simulink model "Xe_Model_Redo_June_26"  (R2018a)
settings: Solver=VariableStepAuto  StartTime=0.0  StopTime=5E5+96*60*60  RelTol=1e-3
values from neighbouring files (symbols this model uses):
  A_pipe = pi*r_pipe^2    (= 0.0126676869774)    [Startup_Script.m]
  alpha_FS = 0.517E-16    (= 5.17e-17)    [Startup_Script.m]
  alpha_G_R1 = 0.334E-17    (= 3.34e-18)    [Startup_Script.m]
  alpha_G_R2 = 0.699E-17    (= 6.99e-18)    [Startup_Script.m]
  alpha_G_R3 = 0.669E-17    (= 6.69e-18)    [Startup_Script.m]
  alpha_G_R4 = 0.791E-18    (= 7.91e-19)    [Startup_Script.m]
  D_g = 2.37E-9    (= 2.37e-09)    [Startup_Script.m]
  epsilon = 0.1    [Startup_Script.m]
  eta_b = 1E-4    (= 0.0001)    [Startup_Script.m]
  eta_fs = 1.2E-4    (= 0.00012)    [Startup_Script.m]
  f_cv = 0.004    [Startup_Script.m]
  FS_Mu_A = 4340    [Startup_Script.m]
  FS_Mu_K = 0.084    [Startup_Script.m]
  FS_Mu_MSRE = 0.007027    [Startup_Script.m]
  FS_rho_A = 3.628    [Startup_Script.m]
  FS_rho_B = 0.00066    [Startup_Script.m]
  FS_rho_MSRE = 2082    [Startup_Script.m]
  gamma_i = 0.0293524    [Startup_Script.m]
  gamma_te = 0.0322482    [Startup_Script.m]
  gamma_xe = 0.00257324    [Startup_Script.m]
  h_fc = 1.6    [Startup_Script.m]
  H_Xe_a = 5.713e-13    [Startup_Script.m]
  H_Xe_b = -7.937e-10    [Startup_Script.m]
  H_Xe_c = 2.809e-07    [Startup_Script.m]
  HX_r_Tube = ((0.5-0.042)/2)*2.54E-2    (= 0.0058166)    [Startup_Script.m]
  HX_XS = HX_N_Tubes*(pi*HX_r_Tube^2)    (= 0.0168999490356)    [Startup_Script.m]
  k_b = 1.3806E-23    (= 1.3806e-23)    [Startup_Script.m]
  lambda_i = 2.9306070546251702E-5    (= 2.93060705463e-05)    [Startup_Script.m]
  lambda_te = 0.036481430555786593    (= 0.0364814305558)    [Startup_Script.m]
  lambda_xe = 2.0924e-05    [Startup_Script.m]
  N_FC_R1 = 12    [Startup_Script.m]
  N_FC_R2 = 940    [Startup_Script.m]
  N_FC_R3 = 108    [Startup_Script.m]
  N_FC_R4 = 78    [Startup_Script.m]
  P_pump = 35420    [Startup_Script.m]
  phi0 = 3.98E+17    (= 3.98e+17)    [Startup_Script.m]
  phi_G_R_1 = mean(interp1(phi_G_R,phi_G_phi, linspace(0,r_g_r1)))    [Startup_Script.m]
  phi_G_R_2 = mean(interp1(phi_G_R,phi_G_phi, linspace(r_g_r1,r_g_r2)))    [Startup_Script.m]
  phi_G_R_3 = mean(interp1(phi_G_R,phi_G_phi, linspace(r_g_r2,r_g_r3)))    [Startup_Script.m]
  phi_G_R_4 = mean(interp1(phi_G_R,phi_G_phi, linspace(r_g_r3,r_g_r4)))    [Startup_Script.m]
  Q_strpr = 0.003155    [Startup_Script.m]
  Q_tot = 0.07571    [Startup_Script.m]
  r_b = 0.000254    [Startup_Script.m]
  r_fc = 0.79e-2    (= 0.0079)    [Startup_Script.m]
  r_pipe = (5E-2*2.54)/2    (= 0.0635)    [Startup_Script.m]
  r_xe = 2.16E-10    (= 2.16e-10)    [Startup_Script.m]
  Re_CA = 25800    [Startup_Script.m]
  Re_LH = 1E4    (= 10000)    [Startup_Script.m]
  Re_UH = 1E4    (= 10000)    [Startup_Script.m]
  sig_a_xe = 1.18E-22    (= 1.18e-22)    [Startup_Script.m]
  Sig_f = 0.15    [Startup_Script.m]
  T_CA_0 = T_INLET    (= 907.594444444)    [Startup_Script.m]
  T_FP_0 = T_OUTLET    (= 935.372222222)    [Startup_Script.m]
  T_FS_R_1_0 = mean(interp1(R_fs_m,T_fs_K, linspace(0,r_g_r1)))    [Startup_Script.m]
  T_FS_R_2_0 = mean(interp1(R_fs_m,T_fs_K, linspace(r_g_r1,r_g_r2)))    [Startup_Script.m]
  T_FS_R_3_0 = mean(interp1(R_fs_m,T_fs_K, linspace(r_g_r2,r_g_r3)))    [Startup_Script.m]
  T_FS_R_4_0 = mean(interp1(R_fs_m,T_fs_K, linspace(r_g_r3,r_g_r4)))    [Startup_Script.m]
  T_G_R_1_0 = mean(interp1(R_gr_m,T_gr_K, linspace(0,r_g_r1)))    [Startup_Script.m]
  T_HX_0 = 0.5*(T_OUTLET + T_INLET)    (= 921.483333333)    [Startup_Script.m]
  T_LH_0 = T_INLET    (= 907.594444444)    [Startup_Script.m]
  T_Mes = 928.15    [Startup_Script.m]
  T_P100_0 = T_OUTLET    (= 935.372222222)    [Startup_Script.m]
  T_P101_0 = T_OUTLET    (= 935.372222222)    [Startup_Script.m]
  T_P102_0 = T_INLET    (= 907.594444444)    [Startup_Script.m]
  T_Salt_0 = 900    [Startup_Script.m]
  T_UH_0 = T_OUTLET    (= 935.372222222)    [Startup_Script.m]
  U_FC_R1 = 0.607    [Startup_Script.m]
  U_FC_R2 = 0.183    [Startup_Script.m]
  U_FC_R3 = 0.454    [Startup_Script.m]
  U_FC_R4 = 0.250    (= 0.25)    [Startup_Script.m]
  V_CA_0 = 9.7*cubed_foot_to_cubed_meter    (= 0.274673445)    [Startup_Script.m]
  V_FP_0 = (0.9+3.2)*cubed_foot_to_cubed_meter    (= 0.116099085)    [Startup_Script.m]
  V_HX_0 = 6.1*cubed_foot_to_cubed_meter    (= 0.172732785)    [Startup_Script.m]
  V_LH_0 = 10.0*cubed_foot_to_cubed_meter    (= 0.2831685)    [Startup_Script.m]
  V_P100_0 = 2.1*cubed_foot_to_cubed_meter    (= 0.059465385)    [Startup_Script.m]
  V_P101_0 = 0.8*cubed_foot_to_cubed_meter    (= 0.02265348)    [Startup_Script.m]
  V_P102_0 = 2.2*cubed_foot_to_cubed_meter    (= 0.06229707)    [Startup_Script.m]
  V_R1_0 = V_Core_FS_0 *N_FC_R1/N_FC_tot    (= 0.00753107712766)    [Startup_Script.m]
  V_R2_0 = V_Core_FS_0 *N_FC_R2/N_FC_tot    (= 0.589934375)    [Startup_Script.m]
  V_R3_0 = V_Core_FS_0 *N_FC_R3/N_FC_tot    (= 0.0677796941489)    [Startup_Script.m]
  V_R4_0 = V_Core_FS_0 *N_FC_R4/N_FC_tot    (= 0.0489520013298)    [Startup_Script.m]
  V_UH_0 = 10.5*cubed_foot_to_cubed_meter    (= 0.297326925)    [Startup_Script.m]
undefined symbols (not defined in the file or in its folder): magnitude, V_CA, V_HX, V_P2, V_P3, V_R1, V_R2, V_R3, V_R4, V_UH
libraries: simulink x4, dspindex x4, dspstat3 x4, SignalEditorBlockLib x2
(part 6 of 11)

== system Xe_Model_Redo_June_26/Bubbles/Bubble Mass Transfer/P100/KMA_P100/Pipe Bubble  MTC ==
  note: ORNL-TM-2245 p. 23 - eqn 36
  note: Thermophysical Properties
  U : Inport
  T : Inport  Port=2
  r : Inport  Port=3
  Constant : Constant  Value=0.0096
  Constant1 : Constant  Value=0.913
  Constant2 : Constant  Value=0.346
  Constant4 : Constant
  Density W Scaling1 : Subsystem
  Divide1 : Product  Inputs=*/
  Gain : Gain  Gain=2
  Mass Diffusion Coeffecient [m^2 /s] : Subsystem
  Math Function : Math  Operator=pow  SaturateOnIntegerOverflow=on
  Math Function1 : Math  Operator=pow  SaturateOnIntegerOverflow=on
  Product : Product
  Reynolds Number : Subsystem
  Schmidt Number : Subsystem
  Sherwood Number : Product  Inputs=4
  Viscosity W Scaling1 : Subsystem
  k_m_b : Outport
  wires:
  Constant1/1 -> Math Function/2
  Gain/1 -> Divide1/2, Reynolds Number/4(L)
  Constant2/1 -> Math Function1/2
  [D_FS_Local] -> Divide1/1
  Constant4/1 -> Sherwood Number/3
  Constant/1 -> Sherwood Number/1
  Divide1/1 -> Product/2
  Math Function1/1 -> Sherwood Number/4
  Schmidt Number/1(Sc) -> Math Function1/1
  Math Function/1 -> Sherwood Number/2
  Sherwood Number/1 -> Product/1
  Product/1 -> k_m_b/1
  Reynolds Number/1(Re) -> Math Function/1
  U/1 -> Reynolds Number/1(Flow_Velocity)
  [Mu_FS_Local] -> Schmidt Number/1(mu)
  [Rho_FS_Local] -> Schmidt Number/2(rho)
  [D_FS_Local] -> Schmidt Number/3(D)
  [Mu_FS_Local] -> Reynolds Number/2(mu)
  [Rho_FS_Local] -> Reynolds Number/3(rho)
  r/1 -> Gain/1
  T/1 -> Mass Diffusion Coeffecient [m^2 /s]/2(T_Salt [k]), Viscosity W Scaling1/1(T_Salt [k]), Density W Scaling1/1(T_Salt [k])
  Density W Scaling1/1(rho_FS [kg/m^3]) -> [Rho_FS_Local]
  Viscosity W Scaling1/1(mu [Pa-s]) -> Mass Diffusion Coeffecient [m^2 /s]/1(Mu), [Mu_FS_Local]
  Mass Diffusion Coeffecient [m^2 /s]/1(D [m^2/s]) -> [D_FS_Local]

== system Xe_Model_Redo_June_26/Bubbles/Bubble Mass Transfer/P101/HRT*C_B /Calc H_Xe ==
  T_Salt [K] : Inport
  Constant : Constant  Value=H_Xe_c
  Math Function : Math  Operator=magnitude^2  SaturateOnIntegerOverflow=on
  Sum1 : Sum  Inputs=+++
  a const : Gain  Gain=H_Xe_a
  b const : Gain  Gain=H_Xe_b
  H_Xe [m^-3 Pa^-1] : Outport
  wires:
  Sum1/1 -> H_Xe [m^-3 Pa^-1]/1
  a const/1 -> Sum1/1
  Constant/1 -> Sum1/3
  b const/1 -> Sum1/2
  Math Function/1 -> a const/1
  T_Salt [K]/1 -> b const/1, Math Function/1

== system Xe_Model_Redo_June_26/Bubbles/Bubble Mass Transfer/P101/KMA_P101/CA  CV Area ==
  Node Vol. : Inport
  CV Vol to Mass Transfer Area1 : Subsystem
  A : Outport
  wires:
  CV Vol to Mass Transfer Area1/1(A) -> A/1
  Node Vol./1 -> CV Vol to Mass Transfer Area1/1(V)

== system Xe_Model_Redo_June_26/Bubbles/Bubble Mass Transfer/P101/KMA_P101/Pipe Bubble  MTC ==
  note: ORNL-TM-2245 p. 23 - eqn 36
  note: Thermophysical Properties
  U : Inport
  T : Inport  Port=2
  r : Inport  Port=3
  Constant : Constant  Value=0.0096
  Constant1 : Constant  Value=0.913
  Constant2 : Constant  Value=0.346
  Constant4 : Constant
  Density W Scaling1 : Subsystem
  Divide1 : Product  Inputs=*/
  Gain : Gain  Gain=2
  Mass Diffusion Coeffecient [m^2 /s] : Subsystem
  Math Function : Math  Operator=pow  SaturateOnIntegerOverflow=on
  Math Function1 : Math  Operator=pow  SaturateOnIntegerOverflow=on
  Product : Product
  Reynolds Number : Subsystem
  Schmidt Number : Subsystem
  Sherwood Number : Product  Inputs=4
  Viscosity W Scaling1 : Subsystem
  k_m_b : Outport
  wires:
  Constant1/1 -> Math Function/2
  r/1 -> Gain/1
  Constant2/1 -> Math Function1/2
  [D_FS_Local] -> Divide1/1
  Constant4/1 -> Sherwood Number/3
  Constant/1 -> Sherwood Number/1
  Divide1/1 -> Product/2
  Math Function1/1 -> Sherwood Number/4
  Schmidt Number/1(Sc) -> Math Function1/1
  Math Function/1 -> Sherwood Number/2
  Sherwood Number/1 -> Product/1
  Product/1 -> k_m_b/1
  Reynolds Number/1(Re) -> Math Function/1
  U/1 -> Reynolds Number/1(Flow_Velocity)
  [Mu_FS_Local] -> Schmidt Number/1(mu)
  [Rho_FS_Local] -> Schmidt Number/2(rho)
  [D_FS_Local] -> Schmidt Number/3(D)
  [Mu_FS_Local] -> Reynolds Number/2(mu)
  [Rho_FS_Local] -> Reynolds Number/3(rho)
  T/1 -> Mass Diffusion Coeffecient [m^2 /s]/2(T_Salt [k]), Viscosity W Scaling1/1(T_Salt [k]), Density W Scaling1/1(T_Salt [k])
  Density W Scaling1/1(rho_FS [kg/m^3]) -> [Rho_FS_Local]
  Viscosity W Scaling1/1(mu [Pa-s]) -> Mass Diffusion Coeffecient [m^2 /s]/1(Mu), [Mu_FS_Local]
  Mass Diffusion Coeffecient [m^2 /s]/1(D [m^2/s]) -> [D_FS_Local]
  Gain/1 -> Divide1/2, Reynolds Number/4(L)

== system Xe_Model_Redo_June_26/Bubbles/Bubble Mass Transfer/P102/HRT*C_B /Calc H_Xe ==
  T_Salt [K] : Inport
  Constant : Constant  Value=H_Xe_c
  Math Function : Math  Operator=magnitude^2  SaturateOnIntegerOverflow=on
  Sum1 : Sum  Inputs=+++
  a const : Gain  Gain=H_Xe_a
  b const : Gain  Gain=H_Xe_b
  H_Xe [m^-3 Pa^-1] : Outport
  wires:
  Sum1/1 -> H_Xe [m^-3 Pa^-1]/1
  a const/1 -> Sum1/1
  Constant/1 -> Sum1/3
  b const/1 -> Sum1/2
  Math Function/1 -> a const/1
  T_Salt [K]/1 -> b const/1, Math Function/1

== system Xe_Model_Redo_June_26/Bubbles/Bubble Mass Transfer/P102/KMA_P102/CA  CV Area ==
  Node Vol. : Inport
  CV Vol to Mass Transfer Area1 : Subsystem
  A : Outport
  wires:
  CV Vol to Mass Transfer Area1/1(A) -> A/1
  Node Vol./1 -> CV Vol to Mass Transfer Area1/1(V)

== system Xe_Model_Redo_June_26/Bubbles/Bubble Mass Transfer/P102/KMA_P102/Pipe Bubble  MTC ==
  note: NB: this is supposed to be for the pipe
  note: ORNL-TM-2245 p. 23 - eqn 36
  note: Thermophysical Properties
  U : Inport
  T : Inport  Port=2
  r : Inport  Port=3
  Constant : Constant  Value=0.0096
  Constant1 : Constant  Value=0.913
  Constant2 : Constant  Value=0.346
  Constant4 : Constant
  Density W Scaling1 : Subsystem
  Divide1 : Product  Inputs=*/
  Gain : Gain  Gain=2
  Mass Diffusion Coeffecient [m^2 /s] : Subsystem
  Math Function : Math  Operator=pow  SaturateOnIntegerOverflow=on
  Math Function1 : Math  Operator=pow  SaturateOnIntegerOverflow=on
  Product : Product
  Reynolds Number : Subsystem
  Schmidt Number : Subsystem
  Sherwood Number : Product  Inputs=4
  Viscosity W Scaling1 : Subsystem
  k_m_b : Outport
  wires:
  Constant1/1 -> Math Function/2
  r/1 -> Gain/1
  Constant2/1 -> Math Function1/2
  [D_FS_Local] -> Divide1/1
  Constant4/1 -> Sherwood Number/3
  Constant/1 -> Sherwood Number/1
  Divide1/1 -> Product/2
  Math Function1/1 -> Sherwood Number/4
  Schmidt Number/1(Sc) -> Math Function1/1
  Math Function/1 -> Sherwood Number/2
  Sherwood Number/1 -> Product/1
  Product/1 -> k_m_b/1
  Reynolds Number/1(Re) -> Math Function/1
  U/1 -> Reynolds Number/1(Flow_Velocity)
  [Mu_FS_Local] -> Schmidt Number/1(mu)
  [Rho_FS_Local] -> Schmidt Number/2(rho)
  [D_FS_Local] -> Schmidt Number/3(D)
  [Mu_FS_Local] -> Reynolds Number/2(mu)
  [Rho_FS_Local] -> Reynolds Number/3(rho)
  T/1 -> Mass Diffusion Coeffecient [m^2 /s]/2(T_Salt [k]), Viscosity W Scaling1/1(T_Salt [k]), Density W Scaling1/1(T_Salt [k])
  Density W Scaling1/1(rho_FS [kg/m^3]) -> [Rho_FS_Local]
  Viscosity W Scaling1/1(mu [Pa-s]) -> Mass Diffusion Coeffecient [m^2 /s]/1(Mu), [Mu_FS_Local]
  Mass Diffusion Coeffecient [m^2 /s]/1(D [m^2/s]) -> [D_FS_Local]
  Gain/1 -> Divide1/2, Reynolds Number/4(L)

== system Xe_Model_Redo_June_26/Bubbles/Bubble Mass Transfer/UH/HRT*C_B /Calc H_Xe ==
  T_Salt [K] : Inport
  Constant : Constant  Value=H_Xe_c
  Math Function : Math  Operator=magnitude^2  SaturateOnIntegerOverflow=on
  Sum1 : Sum  Inputs=+++
  a const : Gain  Gain=H_Xe_a
  b const : Gain  Gain=H_Xe_b
  H_Xe [m^-3 Pa^-1] : Outport
  wires:
  Sum1/1 -> H_Xe [m^-3 Pa^-1]/1
  a const/1 -> Sum1/1
  Constant/1 -> Sum1/3
  b const/1 -> Sum1/2
  Math Function/1 -> a const/1
  T_Salt [K]/1 -> b const/1, Math Function/1

== system Xe_Model_Redo_June_26/Bubbles/Bubble Mass Transfer/UH/KMA_UH/CA  CV Area ==
  Node Vol. : Inport
  CV Vol to Mass Transfer Area1 : Subsystem
  A : Outport
  wires:
  CV Vol to Mass Transfer Area1/1(A) -> A/1
  Node Vol./1 -> CV Vol to Mass Transfer Area1/1(V)

== system Xe_Model_Redo_June_26/Bubbles/Bubble Mass Transfer/UH/KMA_UH/MTC UH ==
  note: Perry's P. 5-69
  note: Thermophysical Properties
  T : Inport
  Constant : Constant  Value=1.0
  Constant1 : Constant  Value=1/3
  Constant2 : Constant  Value=1/3
  Constant3 : Constant  Value=Re_UH
  Constant4 : Constant
  Density W Scaling1 : Subsystem
  Divide1 : Product  Inputs=*/
  Gain : Gain  Gain=2
  Mass Diffusion Coeffecient [m^2 /s]1 : Subsystem
  Math Function : Math  Operator=pow  SaturateOnIntegerOverflow=on
  Math Function1 : Math  Operator=pow  SaturateOnIntegerOverflow=on
  Product : Product
  Re_Num  Scaled : Subsystem
  Schmidt Number : Subsystem
  Sherwood Number : Product  Inputs=4
  Viscosity W Scaling1 : Subsystem
  k_m_b : Outport
  wires:
  Constant1/1 -> Math Function/2
  Constant2/1 -> Math Function1/2
  [D_FS_Local] -> Divide1/1
  Constant4/1 -> Sherwood Number/3
  Constant/1 -> Sherwood Number/1
  Divide1/1 -> Product/2
  Math Function1/1 -> Sherwood Number/4
  Schmidt Number/1(Sc) -> Math Function1/1
  Math Function/1 -> Sherwood Number/2
  Sherwood Number/1 -> Product/1
  Product/1 -> k_m_b/1
  Re_Num  Scaled/1(Re) -> Math Function/1
  [Mu_FS_Local] -> Schmidt Number/1(mu)
  [Rho_FS_Local] -> Schmidt Number/2(rho)
  [D_FS_Local] -> Schmidt Number/3(D)
  T/1 -> Mass Diffusion Coeffecient [m^2 /s]1/2(T_Salt [k]), Viscosity W Scaling1/1(T_Salt [k]), Density W Scaling1/1(T_Salt [k]), Re_Num  Scaled/1(T)
  Density W Scaling1/1(rho_FS [kg/m^3]) -> [Rho_FS_Local]
  Viscosity W Scaling1/1(mu [Pa-s]) -> Mass Diffusion Coeffecient [m^2 /s]1/1(Mu), [Mu_FS_Local]
  Mass Diffusion Coeffecient [m^2 /s]1/1(D [m^2/s]) -> [D_FS_Local]
  Constant3/1 -> Re_Num  Scaled/2(Re_0)
  [r_b] -> Gain/1
  Gain/1 -> Divide1/2

== system Xe_Model_Redo_June_26/Graphite /Graphite Region 1/Graphite MTC R1/Density W Scaling/Cantor F1 Density ==
  note: K -> deg. C
  T_Salt [k] : Inport
  Constant : Constant  Value=FS_rho_A
  Constant1 : Constant  Value=FS_rho_B
  Constant2 : Constant  Value=273.15
  Display : Display
      settings: Format=short_e
  Display1 : Display
  Product : Product
  Sum : Sum  Inputs=|+-
  Sum1 : Sum  Inputs=+-
  "g/cm^3 -> kg/m^3" : Gain  Gain=1000
  rho [kg/m^3] : Outport
  wires:
  Sum/1 -> "g/cm^3 -> kg/m^3"/1
  Product/1 -> Sum/2
  Constant1/1 -> Display/1, Product/1
  "g/cm^3 -> kg/m^3"/1 -> rho [kg/m^3]/1
  Constant/1 -> Display1/1, Sum/1
  T_Salt [k]/1 -> Sum1/1
  Constant2/1 -> Sum1/2
  Sum1/1 -> Product/2

== system Xe_Model_Redo_June_26/Graphite /Graphite Region 1/Graphite MTC R1/Density W Scaling/Cantor F1 Density1 ==
  note: K -> deg. C
  T_Salt [k] : Inport
  Constant : Constant  Value=FS_rho_A
  Constant1 : Constant  Value=FS_rho_B
  Constant2 : Constant  Value=273.15
  Display : Display
      settings: Format=short_e
  Display1 : Display
  Product : Product
  Sum : Sum  Inputs=|+-
  Sum1 : Sum  Inputs=+-
  "g/cm^3 -> kg/m^3" : Gain  Gain=1000
  rho [kg/m^3] : Outport
  wires:
  Sum/1 -> "g/cm^3 -> kg/m^3"/1
  Product/1 -> Sum/2
  Constant1/1 -> Display/1, Product/1
  "g/cm^3 -> kg/m^3"/1 -> rho [kg/m^3]/1
  Constant/1 -> Display1/1, Sum/1
  T_Salt [k]/1 -> Sum1/1
  Constant2/1 -> Sum1/2
  Sum1/1 -> Product/2

== system Xe_Model_Redo_June_26/Graphite /Graphite Region 1/Graphite MTC R1/Viscosity W Scaling/Cantor Viscosity F1 ==
  T_Salt [k] : Inport
  Constant : Constant  Value=FS_Mu_A
  Constant1 : Constant  Value=FS_Mu_K
  Display1 : Display
  Divide : Product  Inputs=*/
  Math Function : Math  SaturateOnIntegerOverflow=on
  Product : Product
  "centipoise -> Pa S" : Gain  Gain=0.001
  Mu [Pa S] : Outport
  wires:
  Constant1/1 -> Product/2
  T_Salt [k]/1 -> Divide/2
  "centipoise -> Pa S"/1 -> Display1/1, Mu [Pa S]/1
  Product/1 -> "centipoise -> Pa S"/1
  Constant/1 -> Divide/1
  Math Function/1 -> Product/1
  Divide/1 -> Math Function/1

== system Xe_Model_Redo_June_26/Graphite /Graphite Region 1/Graphite MTC R1/Viscosity W Scaling/Nominal Value for Cantor Viscosity F1 ==
  T_Salt [k] : Inport
  Constant : Constant  Value=FS_Mu_A
  Constant1 : Constant  Value=FS_Mu_K
  Display1 : Display
  Divide : Product  Inputs=*/
  Math Function : Math  SaturateOnIntegerOverflow=on
  Product : Product
  "centipoise -> Pa S" : Gain  Gain=0.001
  Mu [Pa S] : Outport
  wires:
  Constant1/1 -> Product/2
  T_Salt [k]/1 -> Divide/2
  "centipoise -> Pa S"/1 -> Display1/1, Mu [Pa S]/1
  Product/1 -> "centipoise -> Pa S"/1
  Constant/1 -> Divide/1
  Math Function/1 -> Product/1
  Divide/1 -> Math Function/1

== system Xe_Model_Redo_June_26/Graphite /Graphite Region 1/Graphite Stringer/Calc Flux/Calc H_Xe ==
  T_Salt [K] : Inport
  Constant : Constant  Value=H_Xe_c
  Math Function : Math  Operator=magnitude^2  SaturateOnIntegerOverflow=on
  Sum1 : Sum  Inputs=+++
  a const : Gain  Gain=H_Xe_a
  b const : Gain  Gain=H_Xe_b
  H_Xe [m^-3 Pa^-1] : Outport
  wires:
  Sum1/1 -> H_Xe [m^-3 Pa^-1]/1
  a const/1 -> Sum1/1
  Constant/1 -> Sum1/3
  b const/1 -> Sum1/2
  Math Function/1 -> a const/1
  T_Salt [K]/1 -> b const/1, Math Function/1

== system Xe_Model_Redo_June_26/Graphite /Graphite Region 1/Graphite Stringer/HMat/Calc H_Xe ==
  T_Salt [K] : Inport
  Constant : Constant  Value=H_Xe_c
  Math Function : Math  Operator=magnitude^2  SaturateOnIntegerOverflow=on
  Sum1 : Sum  Inputs=+++
  a const : Gain  Gain=H_Xe_a
  b const : Gain  Gain=H_Xe_b
  H_Xe [m^-3 Pa^-1] : Outport
  wires:
  Sum1/1 -> H_Xe [m^-3 Pa^-1]/1
  a const/1 -> Sum1/1
  Constant/1 -> Sum1/3
  b const/1 -> Sum1/2
  Math Function/1 -> a const/1
  T_Salt [K]/1 -> b const/1, Math Function/1

== system Xe_Model_Redo_June_26/Graphite /Graphite Region 1/Lumped Parameter Graphite Model/Subsystem/HRT over epsilon ==
  T : Inport
  Calc H_Xe : Subsystem
  Divide2 : Product  Inputs=***/
  Out1 : Outport
  wires:
  T/1 -> Calc H_Xe/1(T_Salt [K]), Divide2/3
  [epsilon] -> Divide2/4
  Calc H_Xe/1(H_Xe [m^-3 Pa^-1]) -> Divide2/1
  [R_gas] -> Divide2/2
  Divide2/1 -> Out1/1

== system Xe_Model_Redo_June_26/Graphite /Graphite Region 2/Graphite MTC R1/Density W Scaling/Cantor F1 Density ==
  note: K -> deg. C
  T_Salt [k] : Inport
  Constant : Constant  Value=FS_rho_A
  Constant1 : Constant  Value=FS_rho_B
  Constant2 : Constant  Value=273.15
  Display : Display
      settings: Format=short_e
  Display1 : Display
  Product : Product
  Sum : Sum  Inputs=|+-
  Sum1 : Sum  Inputs=+-
  "g/cm^3 -> kg/m^3" : Gain  Gain=1000
  rho [kg/m^3] : Outport
  wires:
  Sum/1 -> "g/cm^3 -> kg/m^3"/1
  Product/1 -> Sum/2
  Constant1/1 -> Display/1, Product/1
  "g/cm^3 -> kg/m^3"/1 -> rho [kg/m^3]/1
  Constant/1 -> Display1/1, Sum/1
  T_Salt [k]/1 -> Sum1/1
  Constant2/1 -> Sum1/2
  Sum1/1 -> Product/2

== system Xe_Model_Redo_June_26/Graphite /Graphite Region 2/Graphite MTC R1/Density W Scaling/Cantor F1 Density1 ==
  note: K -> deg. C
  T_Salt [k] : Inport
  Constant : Constant  Value=FS_rho_A
  Constant1 : Constant  Value=FS_rho_B
  Constant2 : Constant  Value=273.15
  Display : Display
      settings: Format=short_e
  Display1 : Display
  Product : Product
  Sum : Sum  Inputs=|+-
  Sum1 : Sum  Inputs=+-
  "g/cm^3 -> kg/m^3" : Gain  Gain=1000
  rho [kg/m^3] : Outport
  wires:
  Sum/1 -> "g/cm^3 -> kg/m^3"/1
  Product/1 -> Sum/2
  Constant1/1 -> Display/1, Product/1
  "g/cm^3 -> kg/m^3"/1 -> rho [kg/m^3]/1
  Constant/1 -> Display1/1, Sum/1
  T_Salt [k]/1 -> Sum1/1
  Constant2/1 -> Sum1/2
  Sum1/1 -> Product/2

== system Xe_Model_Redo_June_26/Graphite /Graphite Region 2/Graphite MTC R1/Viscosity W Scaling/Cantor Viscosity F1 ==
  T_Salt [k] : Inport
  Constant : Constant  Value=FS_Mu_A
  Constant1 : Constant  Value=FS_Mu_K
  Display1 : Display
  Divide : Product  Inputs=*/
  Math Function : Math  SaturateOnIntegerOverflow=on
  Product : Product
  "centipoise -> Pa S" : Gain  Gain=0.001
  Mu [Pa S] : Outport
  wires:
  Constant1/1 -> Product/2
  T_Salt [k]/1 -> Divide/2
  "centipoise -> Pa S"/1 -> Display1/1, Mu [Pa S]/1
  Product/1 -> "centipoise -> Pa S"/1
  Constant/1 -> Divide/1
  Math Function/1 -> Product/1
  Divide/1 -> Math Function/1

== system Xe_Model_Redo_June_26/Graphite /Graphite Region 2/Graphite MTC R1/Viscosity W Scaling/Nominal Value for Cantor Viscosity F1 ==
  T_Salt [k] : Inport
  Constant : Constant  Value=FS_Mu_A
  Constant1 : Constant  Value=FS_Mu_K
  Display1 : Display
  Divide : Product  Inputs=*/
  Math Function : Math  SaturateOnIntegerOverflow=on
  Product : Product
  "centipoise -> Pa S" : Gain  Gain=0.001
  Mu [Pa S] : Outport
  wires:
  Constant1/1 -> Product/2
  T_Salt [k]/1 -> Divide/2
  "centipoise -> Pa S"/1 -> Display1/1, Mu [Pa S]/1
  Product/1 -> "centipoise -> Pa S"/1
  Constant/1 -> Divide/1
  Math Function/1 -> Product/1
  Divide/1 -> Math Function/1

== system Xe_Model_Redo_June_26/Graphite /Graphite Region 2/Graphite Stringer/Calc Flux/Calc H_Xe ==
  T_Salt [K] : Inport
  Constant : Constant  Value=H_Xe_c
  Math Function : Math  Operator=magnitude^2  SaturateOnIntegerOverflow=on
  Sum1 : Sum  Inputs=+++
  a const : Gain  Gain=H_Xe_a
  b const : Gain  Gain=H_Xe_b
  H_Xe [m^-3 Pa^-1] : Outport
  wires:
  Sum1/1 -> H_Xe [m^-3 Pa^-1]/1
  a const/1 -> Sum1/1
  Constant/1 -> Sum1/3
  b const/1 -> Sum1/2
  Math Function/1 -> a const/1
  T_Salt [K]/1 -> b const/1, Math Function/1

== system Xe_Model_Redo_June_26/Graphite /Graphite Region 2/Graphite Stringer/HMat/Calc H_Xe ==
  T_Salt [K] : Inport
  Constant : Constant  Value=H_Xe_c
  Math Function : Math  Operator=magnitude^2  SaturateOnIntegerOverflow=on
  Sum1 : Sum  Inputs=+++
  a const : Gain  Gain=H_Xe_a
  b const : Gain  Gain=H_Xe_b
  H_Xe [m^-3 Pa^-1] : Outport
  wires:
  Sum1/1 -> H_Xe [m^-3 Pa^-1]/1
  a const/1 -> Sum1/1
  Constant/1 -> Sum1/3
  b const/1 -> Sum1/2
  Math Function/1 -> a const/1
  T_Salt [K]/1 -> b const/1, Math Function/1

== system Xe_Model_Redo_June_26/Graphite /Graphite Region 3/Graphite MTC R1/Density W Scaling/Cantor F1 Density ==
  note: K -> deg. C
  T_Salt [k] : Inport
  Constant : Constant  Value=FS_rho_A
  Constant1 : Constant  Value=FS_rho_B
  Constant2 : Constant  Value=273.15
  Display : Display
      settings: Format=short_e
  Display1 : Display
  Product : Product
  Sum : Sum  Inputs=|+-
  Sum1 : Sum  Inputs=+-
  "g/cm^3 -> kg/m^3" : Gain  Gain=1000
  rho [kg/m^3] : Outport
  wires:
  Sum/1 -> "g/cm^3 -> kg/m^3"/1
  Product/1 -> Sum/2
  Constant1/1 -> Display/1, Product/1
  "g/cm^3 -> kg/m^3"/1 -> rho [kg/m^3]/1
  Constant/1 -> Display1/1, Sum/1
  T_Salt [k]/1 -> Sum1/1
  Constant2/1 -> Sum1/2
  Sum1/1 -> Product/2

== system Xe_Model_Redo_June_26/Graphite /Graphite Region 3/Graphite MTC R1/Density W Scaling/Cantor F1 Density1 ==
  note: K -> deg. C
  T_Salt [k] : Inport
  Constant : Constant  Value=FS_rho_A
  Constant1 : Constant  Value=FS_rho_B
  Constant2 : Constant  Value=273.15
  Display : Display
      settings: Format=short_e
  Display1 : Display
  Product : Product
  Sum : Sum  Inputs=|+-
  Sum1 : Sum  Inputs=+-
  "g/cm^3 -> kg/m^3" : Gain  Gain=1000
  rho [kg/m^3] : Outport
  wires:
  Sum/1 -> "g/cm^3 -> kg/m^3"/1
  Product/1 -> Sum/2
  Constant1/1 -> Display/1, Product/1
  "g/cm^3 -> kg/m^3"/1 -> rho [kg/m^3]/1
  Constant/1 -> Display1/1, Sum/1
  T_Salt [k]/1 -> Sum1/1
  Constant2/1 -> Sum1/2
  Sum1/1 -> Product/2

== system Xe_Model_Redo_June_26/Graphite /Graphite Region 3/Graphite MTC R1/Viscosity W Scaling/Cantor Viscosity F1 ==
  T_Salt [k] : Inport
  Constant : Constant  Value=FS_Mu_A
  Constant1 : Constant  Value=FS_Mu_K
  Display1 : Display
  Divide : Product  Inputs=*/
  Math Function : Math  SaturateOnIntegerOverflow=on
  Product : Product
  "centipoise -> Pa S" : Gain  Gain=0.001
  Mu [Pa S] : Outport
  wires:
  Constant1/1 -> Product/2
  T_Salt [k]/1 -> Divide/2
  "centipoise -> Pa S"/1 -> Display1/1, Mu [Pa S]/1
  Product/1 -> "centipoise -> Pa S"/1
  Constant/1 -> Divide/1
  Math Function/1 -> Product/1
  Divide/1 -> Math Function/1

== system Xe_Model_Redo_June_26/Graphite /Graphite Region 3/Graphite MTC R1/Viscosity W Scaling/Nominal Value for Cantor Viscosity F1 ==
  T_Salt [k] : Inport
  Constant : Constant  Value=FS_Mu_A
  Constant1 : Constant  Value=FS_Mu_K
  Display1 : Display
  Divide : Product  Inputs=*/
  Math Function : Math  SaturateOnIntegerOverflow=on
  Product : Product
  "centipoise -> Pa S" : Gain  Gain=0.001
  Mu [Pa S] : Outport
  wires:
  Constant1/1 -> Product/2
  T_Salt [k]/1 -> Divide/2
  "centipoise -> Pa S"/1 -> Display1/1, Mu [Pa S]/1
  Product/1 -> "centipoise -> Pa S"/1
  Constant/1 -> Divide/1
  Math Function/1 -> Product/1
  Divide/1 -> Math Function/1

== system Xe_Model_Redo_June_26/Graphite /Graphite Region 3/Graphite Stringer/Calc Flux/Calc H_Xe ==
  T_Salt [K] : Inport
  Constant : Constant  Value=H_Xe_c
  Math Function : Math  Operator=magnitude^2  SaturateOnIntegerOverflow=on
  Sum1 : Sum  Inputs=+++
  a const : Gain  Gain=H_Xe_a
  b const : Gain  Gain=H_Xe_b
  H_Xe [m^-3 Pa^-1] : Outport
  wires:
  Sum1/1 -> H_Xe [m^-3 Pa^-1]/1
  a const/1 -> Sum1/1
  Constant/1 -> Sum1/3
  b const/1 -> Sum1/2
  Math Function/1 -> a const/1
  T_Salt [K]/1 -> b const/1, Math Function/1

== system Xe_Model_Redo_June_26/Graphite /Graphite Region 3/Graphite Stringer/HMat/Calc H_Xe ==
  T_Salt [K] : Inport
  Constant : Constant  Value=H_Xe_c
  Math Function : Math  Operator=magnitude^2  SaturateOnIntegerOverflow=on
  Sum1 : Sum  Inputs=+++
  a const : Gain  Gain=H_Xe_a
  b const : Gain  Gain=H_Xe_b
  H_Xe [m^-3 Pa^-1] : Outport
  wires:
  Sum1/1 -> H_Xe [m^-3 Pa^-1]/1
  a const/1 -> Sum1/1
  Constant/1 -> Sum1/3
  b const/1 -> Sum1/2
  Math Function/1 -> a const/1
  T_Salt [K]/1 -> b const/1, Math Function/1

== system Xe_Model_Redo_June_26/Graphite /Graphite Region 4/Graphite MTC R1/Density W Scaling/Cantor F1 Density ==
  note: K -> deg. C
  T_Salt [k] : Inport
  Constant : Constant  Value=FS_rho_A
  Constant1 : Constant  Value=FS_rho_B
  Constant2 : Constant  Value=273.15
  Display : Display
      settings: Format=short_e
  Display1 : Display
  Product : Product
  Sum : Sum  Inputs=|+-
  Sum1 : Sum  Inputs=+-
  "g/cm^3 -> kg/m^3" : Gain  Gain=1000
  rho [kg/m^3] : Outport
  wires:
  Sum/1 -> "g/cm^3 -> kg/m^3"/1
  Product/1 -> Sum/2
  Constant1/1 -> Display/1, Product/1
  "g/cm^3 -> kg/m^3"/1 -> rho [kg/m^3]/1
  Constant/1 -> Display1/1, Sum/1
  T_Salt [k]/1 -> Sum1/1
  Constant2/1 -> Sum1/2
  Sum1/1 -> Product/2

== system Xe_Model_Redo_June_26/Graphite /Graphite Region 4/Graphite MTC R1/Density W Scaling/Cantor F1 Density1 ==
  note: K -> deg. C
  T_Salt [k] : Inport
  Constant : Constant  Value=FS_rho_A
  Constant1 : Constant  Value=FS_rho_B
  Constant2 : Constant  Value=273.15
  Display : Display
      settings: Format=short_e
  Display1 : Display
  Product : Product
  Sum : Sum  Inputs=|+-
  Sum1 : Sum  Inputs=+-
  "g/cm^3 -> kg/m^3" : Gain  Gain=1000
  rho [kg/m^3] : Outport
  wires:
  Sum/1 -> "g/cm^3 -> kg/m^3"/1
  Product/1 -> Sum/2
  Constant1/1 -> Display/1, Product/1
  "g/cm^3 -> kg/m^3"/1 -> rho [kg/m^3]/1
  Constant/1 -> Display1/1, Sum/1
  T_Salt [k]/1 -> Sum1/1
  Constant2/1 -> Sum1/2
  Sum1/1 -> Product/2

== system Xe_Model_Redo_June_26/Graphite /Graphite Region 4/Graphite MTC R1/Viscosity W Scaling/Cantor Viscosity F1 ==
  T_Salt [k] : Inport
  Constant : Constant  Value=FS_Mu_A
  Constant1 : Constant  Value=FS_Mu_K
  Display1 : Display
  Divide : Product  Inputs=*/
  Math Function : Math  SaturateOnIntegerOverflow=on
  Product : Product
  "centipoise -> Pa S" : Gain  Gain=0.001
  Mu [Pa S] : Outport
  wires:
  Constant1/1 -> Product/2
  T_Salt [k]/1 -> Divide/2
  "centipoise -> Pa S"/1 -> Display1/1, Mu [Pa S]/1
  Product/1 -> "centipoise -> Pa S"/1
  Constant/1 -> Divide/1
  Math Function/1 -> Product/1
  Divide/1 -> Math Function/1

== system Xe_Model_Redo_June_26/Graphite /Graphite Region 4/Graphite MTC R1/Viscosity W Scaling/Nominal Value for Cantor Viscosity F1 ==
  T_Salt [k] : Inport
  Constant : Constant  Value=FS_Mu_A
  Constant1 : Constant  Value=FS_Mu_K
  Display1 : Display
  Divide : Product  Inputs=*/
  Math Function : Math  SaturateOnIntegerOverflow=on
  Product : Product
  "centipoise -> Pa S" : Gain  Gain=0.001
  Mu [Pa S] : Outport
  wires:
  Constant1/1 -> Product/2
  T_Salt [k]/1 -> Divide/2
  "centipoise -> Pa S"/1 -> Display1/1, Mu [Pa S]/1
  Product/1 -> "centipoise -> Pa S"/1
  Constant/1 -> Divide/1
  Math Function/1 -> Product/1
  Divide/1 -> Math Function/1

== system Xe_Model_Redo_June_26/Graphite /Graphite Region 4/Graphite Stringer/Calc Flux/Calc H_Xe ==
  T_Salt [K] : Inport
  Constant : Constant  Value=H_Xe_c
  Math Function : Math  Operator=magnitude^2  SaturateOnIntegerOverflow=on
  Sum1 : Sum  Inputs=+++
  a const : Gain  Gain=H_Xe_a
  b const : Gain  Gain=H_Xe_b
  H_Xe [m^-3 Pa^-1] : Outport
  wires:
  Sum1/1 -> H_Xe [m^-3 Pa^-1]/1
  a const/1 -> Sum1/1
  Constant/1 -> Sum1/3
  b const/1 -> Sum1/2
  Math Function/1 -> a const/1
  T_Salt [K]/1 -> b const/1, Math Function/1

== system Xe_Model_Redo_June_26/Graphite /Graphite Region 4/Graphite Stringer/HMat/Calc H_Xe ==
  T_Salt [K] : Inport
  Constant : Constant  Value=H_Xe_c
  Math Function : Math  Operator=magnitude^2  SaturateOnIntegerOverflow=on
  Sum1 : Sum  Inputs=+++
  a const : Gain  Gain=H_Xe_a
  b const : Gain  Gain=H_Xe_b
  H_Xe [m^-3 Pa^-1] : Outport
  wires:
  Sum1/1 -> H_Xe [m^-3 Pa^-1]/1
  a const/1 -> Sum1/1
  Constant/1 -> Sum1/3
  b const/1 -> Sum1/2
  Math Function/1 -> a const/1
  T_Salt [K]/1 -> b const/1, Math Function/1

== system Xe_Model_Redo_June_26/Bubbles/Bubble Mass Transfer/Bubble Total KMA/HX KMA/CA  CV Area/CV Vol to Mass Transfer Area1 ==
  V : Inport
  Divide1 : Product  Inputs=*/
  Product3 : Product
  A : Outport
  wires:
  V/1 -> Divide1/1
  Divide1/1 -> Product3/2
  [V_1_B] -> Divide1/2
  [A_1_B] -> Product3/1
  Product3/1 -> A/1

== system Xe_Model_Redo_June_26/Bubbles/Bubble Mass Transfer/Bubble Total KMA/HX KMA/CA  CV Area/Calc CV Vol W Temp ==
  note: Total CV Vol
  Vol. Gas : Inport
  T : Inport  Port=2
  Constant1 : Constant  Value=T_Salt_0
  Divide : Product  Inputs=**/
  Product : Product
  Product1 : Product
  Subtract1 : Sum  Inputs=+-
  Sum1 : Sum
  vol to num atoms1 : Subsystem
  V Gas : Outport
  wires:
  Product/1 -> Sum1/1, vol to num atoms1/1(vol)
  vol to num atoms1/1(N mols) -> Divide/1
  Product1/1 -> Sum1/2
  T/1 -> Subtract1/1
  Constant1/1 -> Subtract1/2
  Sum1/1 -> V Gas/1
  Vol. Gas/1 -> Product/2
  [R_gas] -> Divide/2
  [P_sys] -> Divide/3
  Divide/1 -> Product1/1
  Subtract1/1 -> Product1/2
  [f_cv_0] -> Product/1

== system Xe_Model_Redo_June_26/Bubbles/Bubble Mass Transfer/Bubble Total KMA/HX KMA/Pipe Buble MTC1/Density W Scaling1 ==
  T_Salt [k] : Inport
  Cantor F1 Density : Subsystem
  Cantor F1 Density1 : Subsystem
  Constant3 : Constant  Value=T_Mes
  Constant4 : Constant  Value=FS_rho_MSRE
  Divide1 : Product  Inputs=*/
  Product1 : Product
  rho_FS [kg/m^3] : Outport
  wires:
  Divide1/1 -> Product1/2
  Cantor F1 Density1/1(rho [kg/m^3]) -> Divide1/2
  Constant4/1 -> Product1/1
  Cantor F1 Density/1(rho [kg/m^3]) -> Divide1/1
  Product1/1 -> rho_FS [kg/m^3]/1
  Constant3/1 -> Cantor F1 Density1/1(T_Salt [k])
  T_Salt [k]/1 -> Cantor F1 Density/1(T_Salt [k])

== system Xe_Model_Redo_June_26/Bubbles/Bubble Mass Transfer/Bubble Total KMA/HX KMA/Pipe Buble MTC1/Mass Diffusion Coeffecient [m^2 //s] ==
  Mu : Inport
  T_Salt [k] : Inport  Port=2
  Constant : Constant  Value=k_b
  Constant1 : Constant  Value=6*pi
  Constant2 : Constant  Value=r_xe
  Divide : Product  Inputs=*/
  Product : Product
  Product1 : Product  Inputs=3
  D [m^2/s] : Outport
  wires:
  Constant1/1 -> Product1/1
  Constant2/1 -> Product1/3
  T_Salt [k]/1 -> Product/1
  Product1/1 -> Divide/2
  Constant/1 -> Product/2
  Product/1 -> Divide/1
  Divide/1 -> D [m^2/s]/1
  Mu/1 -> Product1/2

== system Xe_Model_Redo_June_26/Bubbles/Bubble Mass Transfer/Bubble Total KMA/HX KMA/Pipe Buble MTC1/Reynolds Number ==
  Flow_Velocity : Inport
  mu : Inport  Port=2
  rho : Inport  Port=3
  L : Inport  Port=4
  Divide : Product  Inputs=***/
  Re : Outport
  wires:
  mu/1 -> Divide/4
  rho/1 -> Divide/1
  Divide/1 -> Re/1
  Flow_Velocity/1 -> Divide/2
  L/1 -> Divide/3

== system Xe_Model_Redo_June_26/Bubbles/Bubble Mass Transfer/Bubble Total KMA/HX KMA/Pipe Buble MTC1/Reynolds Number1 ==
  Flow_Velocity [m/s] : Inport
  rho [kg/m^3] : Inport  Port=2
  mu [Pa s] : Inport  Port=3
  Divide : Product  Inputs=***/
  Re : Outport
  wires:
  mu [Pa s]/1 -> Divide/4
  rho [kg/m^3]/1 -> Divide/1
  Divide/1 -> Re/1
  Flow_Velocity [m/s]/1 -> Divide/2
  [r_fc] -> Divide/3

== system Xe_Model_Redo_June_26/Bubbles/Bubble Mass Transfer/Bubble Total KMA/HX KMA/Pipe Buble MTC1/Schmidt Number ==
  mu : Inport
  rho : Inport  Port=2
  D : Inport  Port=3
  Product : Product  Inputs=*//
  Sc : Outport
  wires:
  Product/1 -> Sc/1
  D/1 -> Product/3
  mu/1 -> Product/1
  rho/1 -> Product/2

== system Xe_Model_Redo_June_26/Bubbles/Bubble Mass Transfer/Bubble Total KMA/HX KMA/Pipe Buble MTC1/Schmidt Number1 ==
  mu [Pa s] : Inport
  rho [kg/m^3] : Inport  Port=2
  D [m^2/s] : Inport  Port=3
  Product : Product  Inputs=*//
  Sc : Outport
  wires:
  Product/1 -> Sc/1
  D [m^2/s]/1 -> Product/3
  mu [Pa s]/1 -> Product/1
  rho [kg/m^3]/1 -> Product/2

== system Xe_Model_Redo_June_26/Bubbles/Bubble Mass Transfer/Bubble Total KMA/HX KMA/Pipe Buble MTC1/Viscosity W Scaling1 ==
  T_Salt [k] : Inport
  Cantor Viscosity F1 : Subsystem
  Constant3 : Constant  Value=T_Mes
  Constant4 : Constant  Value=FS_Mu_MSRE
  Divide1 : Product  Inputs=*/
  Nominal Value for Cantor Viscosity F1 : Subsystem
  Product1 : Product
  mu [Pa-s] : Outport
  wires:
  Nominal Value for Cantor Viscosity F1/1(Mu [Pa S]) -> Divide1/2
  Divide1/1 -> Product1/2
  Cantor Viscosity F1/1(Mu [Pa S]) -> Divide1/1
  Product1/1 -> mu [Pa-s]/1
  Constant4/1 -> Product1/1
  Constant3/1 -> Nominal Value for Cantor Viscosity F1/1(T_Salt [k])
  T_Salt [k]/1 -> Cantor Viscosity F1/1(T_Salt [k])

== system Xe_Model_Redo_June_26/Bubbles/Bubble Mass Transfer/Bubble Total KMA/KMA FP/CA  CV Area/CV Vol to Mass Transfer Area1 ==
  V : Inport
  Divide1 : Product  Inputs=*/
  Product3 : Product
  A : Outport
  wires:
  V/1 -> Divide1/1
  Divide1/1 -> Product3/2
  [V_1_B] -> Divide1/2
  [A_1_B] -> Product3/1
  Product3/1 -> A/1

== system Xe_Model_Redo_June_26/Bubbles/Bubble Mass Transfer/Bubble Total KMA/KMA FP/CA  CV Area/Calc CV Vol W Temp ==
  note: Total CV Vol
  Vol. Gas : Inport
  T : Inport  Port=2
  Constant1 : Constant  Value=T_Salt_0
  Divide : Product  Inputs=**/
  Product : Product
  Product1 : Product
  Subtract1 : Sum  Inputs=+-
  Sum1 : Sum
  vol to num atoms1 : Subsystem
  V Gas : Outport
  wires:
  Product/1 -> Sum1/1, vol to num atoms1/1(vol)
  vol to num atoms1/1(N mols) -> Divide/1
  Product1/1 -> Sum1/2
  T/1 -> Subtract1/1
  Constant1/1 -> Subtract1/2
  Sum1/1 -> V Gas/1
  Vol. Gas/1 -> Product/2
  [R_gas] -> Divide/2
  [P_sys] -> Divide/3
  Divide/1 -> Product1/1
  Subtract1/1 -> Product1/2
  [f_cv_0] -> Product/1

== system Xe_Model_Redo_June_26/Bubbles/Bubble Mass Transfer/Bubble Total KMA/KMA FP/Pump Bowl MTC1/Density W Scaling1 ==
  T_Salt [k] : Inport
  Cantor F1 Density : Subsystem
  Cantor F1 Density1 : Subsystem
  Constant3 : Constant  Value=T_Mes
  Constant4 : Constant  Value=FS_rho_MSRE
  Divide1 : Product  Inputs=*/
  Product1 : Product
  rho_FS [kg/m^3] : Outport
  wires:
  Divide1/1 -> Product1/2
  Cantor F1 Density1/1(rho [kg/m^3]) -> Divide1/2
  Constant4/1 -> Product1/1
  Cantor F1 Density/1(rho [kg/m^3]) -> Divide1/1
  Product1/1 -> rho_FS [kg/m^3]/1
  Constant3/1 -> Cantor F1 Density1/1(T_Salt [k])
  T_Salt [k]/1 -> Cantor F1 Density/1(T_Salt [k])

== system Xe_Model_Redo_June_26/Bubbles/Bubble Mass Transfer/Bubble Total KMA/KMA FP/Pump Bowl MTC1/Mass Diffusion Coeffecient [m^2 //s] ==
  Mu : Inport
  T_Salt [k] : Inport  Port=2
  Constant : Constant  Value=k_b
  Constant1 : Constant  Value=6*pi
  Constant2 : Constant  Value=r_xe
  Divide : Product  Inputs=*/
  Product : Product
  Product1 : Product  Inputs=3
  D [m^2/s] : Outport
  wires:
  Constant1/1 -> Product1/1
  Constant2/1 -> Product1/3
  T_Salt [k]/1 -> Product/1
  Product1/1 -> Divide/2
  Constant/1 -> Product/2
  Product/1 -> Divide/1
  Divide/1 -> D [m^2/s]/1
  Mu/1 -> Product1/2

== system Xe_Model_Redo_June_26/Bubbles/Bubble Mass Transfer/Bubble Total KMA/KMA FP/Pump Bowl MTC1/Schmidt Number1 ==
  mu [Pa s] : Inport
  rho [kg/m^3] : Inport  Port=2
  D [m^2/s] : Inport  Port=3
  Product : Product  Inputs=*//
  Sc : Outport
  wires:
  Product/1 -> Sc/1
  D [m^2/s]/1 -> Product/3
  mu [Pa s]/1 -> Product/1
  rho [kg/m^3]/1 -> Product/2

== system Xe_Model_Redo_June_26/Bubbles/Bubble Mass Transfer/Bubble Total KMA/KMA FP/Pump Bowl MTC1/Viscosity W Scaling1 ==
  T_Salt [k] : Inport
  Cantor Viscosity F1 : Subsystem
  Constant3 : Constant  Value=T_Mes
  Constant4 : Constant  Value=FS_Mu_MSRE
  Divide1 : Product  Inputs=*/
  Nominal Value for Cantor Viscosity F1 : Subsystem
  Product1 : Product
  mu [Pa-s] : Outport
  wires:
  Nominal Value for Cantor Viscosity F1/1(Mu [Pa S]) -> Divide1/2
  Divide1/1 -> Product1/2
  Cantor Viscosity F1/1(Mu [Pa S]) -> Divide1/1
  Product1/1 -> mu [Pa-s]/1
  Constant4/1 -> Product1/1
  Constant3/1 -> Nominal Value for Cantor Viscosity F1/1(T_Salt [k])
  T_Salt [k]/1 -> Cantor Viscosity F1/1(T_Salt [k])

== system Xe_Model_Redo_June_26/Bubbles/Bubble Mass Transfer/Bubble Total KMA/KMA_CA/CA  CV Area/CV Vol to Mass Transfer Area1 ==
  V : Inport
  Divide1 : Product  Inputs=*/
  Product3 : Product
  A : Outport
  wires:
  V/1 -> Divide1/1
  Divide1/1 -> Product3/2
  [V_1_B] -> Divide1/2
  [A_1_B] -> Product3/1
  Product3/1 -> A/1

== system Xe_Model_Redo_June_26/Bubbles/Bubble Mass Transfer/Bubble Total KMA/KMA_CA/CA  CV Area/Calc CV Vol W Temp ==
  note: Total CV Vol
  Vol. Gas : Inport
  T : Inport  Port=2
  Constant1 : Constant  Value=T_Salt_0
  Divide : Product  Inputs=**/
  Product : Product
  Product1 : Product
  Subtract1 : Sum  Inputs=+-
  Sum1 : Sum
  vol to num atoms1 : Subsystem
  V Gas : Outport
  wires:
  Product/1 -> Sum1/1, vol to num atoms1/1(vol)
  vol to num atoms1/1(N mols) -> Divide/1
  Product1/1 -> Sum1/2
  T/1 -> Subtract1/1
  Constant1/1 -> Subtract1/2
  Sum1/1 -> V Gas/1
  Vol. Gas/1 -> Product/2
  [R_gas] -> Divide/2
  [P_sys] -> Divide/3
  Divide/1 -> Product1/1
  Subtract1/1 -> Product1/2
  [f_cv_0] -> Product/1

== system Xe_Model_Redo_June_26/Bubbles/Bubble Mass Transfer/Bubble Total KMA/KMA_CA/CA  MTC/Density W Scaling1 ==
  T_Salt [k] : Inport
  Cantor F1 Density : Subsystem
  Cantor F1 Density1 : Subsystem
  Constant3 : Constant  Value=T_Mes
  Constant4 : Constant  Value=FS_rho_MSRE
  Divide1 : Product  Inputs=*/
  Product1 : Product
  rho_FS [kg/m^3] : Outport
  wires:
  Divide1/1 -> Product1/2
  Cantor F1 Density1/1(rho [kg/m^3]) -> Divide1/2
  Constant4/1 -> Product1/1
  Cantor F1 Density/1(rho [kg/m^3]) -> Divide1/1
  Product1/1 -> rho_FS [kg/m^3]/1
  Constant3/1 -> Cantor F1 Density1/1(T_Salt [k])
  T_Salt [k]/1 -> Cantor F1 Density/1(T_Salt [k])

== system Xe_Model_Redo_June_26/Bubbles/Bubble Mass Transfer/Bubble Total KMA/KMA_CA/CA  MTC/Mass Diffusion Coeffecient [m^2 //s] ==
  Mu : Inport
  T_Salt [k] : Inport  Port=2
  Constant : Constant  Value=k_b
  Constant1 : Constant  Value=6*pi
  Constant2 : Constant  Value=r_xe
  Divide : Product  Inputs=*/
  Product : Product
  Product1 : Product  Inputs=3
  D [m^2/s] : Outport
  wires:
  Constant1/1 -> Product1/1
  Constant2/1 -> Product1/3
  T_Salt [k]/1 -> Product/1
  Product1/1 -> Divide/2
  Constant/1 -> Product/2
  Product/1 -> Divide/1
  Divide/1 -> D [m^2/s]/1
  Mu/1 -> Product1/2

== system Xe_Model_Redo_June_26/Bubbles/Bubble Mass Transfer/Bubble Total KMA/KMA_CA/CA  MTC/Re_Num  Scaled ==
  T : Inport
  Re_0 : Inport  Port=2
  Constant1 : Constant  Value=T_Mes
  Density W Scaling1 : Subsystem
  Density W Scaling3 : Subsystem
  Display1 : Display
  Divide1 : Product  Inputs=*/
  Divide2 : Product  Inputs=*/
  Divide3 : Product  Inputs=*/
  Multiply1 : Product
  Viscosity W Scaling1 : Subsystem
  Viscosity W Scaling3 : Subsystem
  Re : Outport
  wires:
  Viscosity W Scaling1/1(mu [Pa-s]) -> Divide1/2
  Constant1/1 -> Viscosity W Scaling1/1(T_Salt [k]), Density W Scaling1/1(T_Salt [k])
  Density W Scaling1/1(rho_FS [kg/m^3]) -> Divide1/1
  T/1 -> Viscosity W Scaling3/1(T_Salt [k]), Density W Scaling3/1(T_Salt [k])
  Density W Scaling3/1(rho_FS [kg/m^3]) -> Divide2/1
  Viscosity W Scaling3/1(mu [Pa-s]) -> Divide2/2
  Divide2/1 -> Divide3/1
  Divide1/1 -> Divide3/2
  Divide3/1 -> Display1/1, Multiply1/1
  Re_0/1 -> Multiply1/2
  Multiply1/1 -> Re/1

== system Xe_Model_Redo_June_26/Bubbles/Bubble Mass Transfer/Bubble Total KMA/KMA_CA/CA  MTC/Schmidt Number ==
  mu : Inport
  rho : Inport  Port=2
  D : Inport  Port=3
  Product : Product  Inputs=*//
  Sc : Outport
  wires:
  Product/1 -> Sc/1
  D/1 -> Product/3
  mu/1 -> Product/1
  rho/1 -> Product/2

== system Xe_Model_Redo_June_26/Bubbles/Bubble Mass Transfer/Bubble Total KMA/KMA_CA/CA  MTC/Viscosity W Scaling1 ==
  T_Salt [k] : Inport
  Cantor Viscosity F1 : Subsystem
  Constant3 : Constant  Value=T_Mes
  Constant4 : Constant  Value=FS_Mu_MSRE
  Divide1 : Product  Inputs=*/
  Nominal Value for Cantor Viscosity F1 : Subsystem
  Product1 : Product
  mu [Pa-s] : Outport
  wires:
  Nominal Value for Cantor Viscosity F1/1(Mu [Pa S]) -> Divide1/2
  Divide1/1 -> Product1/2
  Cantor Viscosity F1/1(Mu [Pa S]) -> Divide1/1
  Product1/1 -> mu [Pa-s]/1
  Constant4/1 -> Product1/1
  Constant3/1 -> Nominal Value for Cantor Viscosity F1/1(T_Salt [k])
  T_Salt [k]/1 -> Cantor Viscosity F1/1(T_Salt [k])

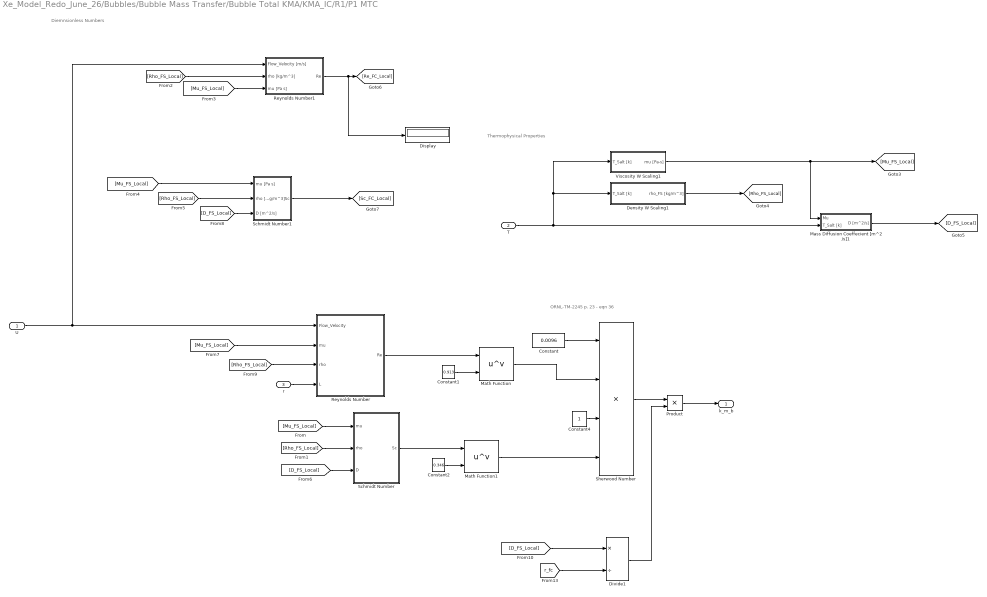
== system Xe_Model_Redo_June_26/Bubbles/Bubble Mass Transfer/Bubble Total KMA/KMA_IC/R1/P1 MTC ==
  note: ORNL-TM-2245 p. 23 - eqn 36
  note: Diemnsionless Numbers
  note: Thermophysical Properties
  U : Inport
  T : Inport  Port=2
  r : Inport  Port=3
  Constant : Constant  Value=0.0096
  Constant1 : Constant  Value=0.913
  Constant2 : Constant  Value=0.346
  Constant4 : Constant
  Density W Scaling1 : Subsystem
  Display : Display
  Divide1 : Product  Inputs=*/
  Mass Diffusion Coeffecient [m^2 /s]1 : Subsystem
  Math Function : Math  Operator=pow  SaturateOnIntegerOverflow=on
  Math Function1 : Math  Operator=pow  SaturateOnIntegerOverflow=on
  Product : Product
  Reynolds Number : Subsystem
  Reynolds Number1 : Subsystem
  Schmidt Number : Subsystem
  Schmidt Number1 : Subsystem
  Sherwood Number : Product  Inputs=4
  Viscosity W Scaling1 : Subsystem
  k_m_b : Outport
  wires:
  Constant1/1 -> Math Function/2
  [r_fc] -> Divide1/2
  Constant2/1 -> Math Function1/2
  [D_FS_Local] -> Divide1/1
  Constant4/1 -> Sherwood Number/3
  Constant/1 -> Sherwood Number/1
  Divide1/1 -> Product/2
  Math Function1/1 -> Sherwood Number/4
  Schmidt Number/1(Sc) -> Math Function1/1
  Math Function/1 -> Sherwood Number/2
  Sherwood Number/1 -> Product/1
  Product/1 -> k_m_b/1
  Reynolds Number/1(Re) -> Math Function/1
  Schmidt Number1/1(Sc) -> [Sc_FC_Local]
  Reynolds Number1/1(Re) -> Display/1, [Re_FC_Local]
  U/1 -> Reynolds Number1/1(Flow_Velocity [m/s]), Reynolds Number/1(Flow_Velocity)
  [Rho_FS_Local] -> Reynolds Number1/2(rho [kg/m^3])
  [Mu_FS_Local] -> Reynolds Number1/3(mu [Pa s])
  [Mu_FS_Local] -> Schmidt Number1/1(mu [Pa s])
  [Rho_FS_Local] -> Schmidt Number1/2(rho [kg/m^3])
  [D_FS_Local] -> Schmidt Number1/3(D [m^2/s])
  [Mu_FS_Local] -> Schmidt Number/1(mu)
  [Rho_FS_Local] -> Schmidt Number/2(rho)
  [D_FS_Local] -> Schmidt Number/3(D)
  [Mu_FS_Local] -> Reynolds Number/2(mu)
  [Rho_FS_Local] -> Reynolds Number/3(rho)
  r/1 -> Reynolds Number/4(L)
  T/1 -> Mass Diffusion Coeffecient [m^2 /s]1/2(T_Salt [k]), Viscosity W Scaling1/1(T_Salt [k]), Density W Scaling1/1(T_Salt [k])
  Density W Scaling1/1(rho_FS [kg/m^3]) -> [Rho_FS_Local]
  Viscosity W Scaling1/1(mu [Pa-s]) -> Mass Diffusion Coeffecient [m^2 /s]1/1(Mu), [Mu_FS_Local]
  Mass Diffusion Coeffecient [m^2 /s]1/1(D [m^2/s]) -> [D_FS_Local]

== system Xe_Model_Redo_June_26/Bubbles/Bubble Mass Transfer/Bubble Total KMA/KMA_IC/R1/R1  CV Area ==
  Node Vol. : Inport
  Node T : Inport  Port=2
  CV Vol to Mass Transfer Area1 : Subsystem
  Calc CV Vol W Temp : Subsystem
  A : Outport
  wires:
  CV Vol to Mass Transfer Area1/1(A) -> A/1
  Node T/1 -> Calc CV Vol W Temp/2(T)
  Node Vol./1 -> Calc CV Vol W Temp/1(Vol. Gas)
  Calc CV Vol W Temp/1(V Gas) -> CV Vol to Mass Transfer Area1/1(V)

== system Xe_Model_Redo_June_26/Bubbles/Bubble Mass Transfer/Bubble Total KMA/KMA_IC/R2/P1 MTC ==
  note: ORNL-TM-2245 p. 23 - eqn 36
  note: Diemnsionless Numbers
  note: Thermophysical Properties
  U : Inport
  T : Inport  Port=2
  r : Inport  Port=3
  Constant : Constant  Value=0.0096
  Constant1 : Constant  Value=0.913
  Constant2 : Constant  Value=0.346
  Constant4 : Constant
  Density W Scaling1 : Subsystem
  Display : Display
  Divide1 : Product  Inputs=*/
  Mass Diffusion Coeffecient [m^2 /s] : Subsystem
  Math Function : Math  Operator=pow  SaturateOnIntegerOverflow=on
  Math Function1 : Math  Operator=pow  SaturateOnIntegerOverflow=on
  Product : Product
  Reynolds Number : Subsystem
  Reynolds Number1 : Subsystem
  Schmidt Number : Subsystem
  Schmidt Number1 : Subsystem
  Sherwood Number : Product  Inputs=4
  Viscosity W Scaling1 : Subsystem
  k_m_b : Outport
  wires:
  Constant1/1 -> Math Function/2
  [r_fc] -> Divide1/2
  Constant2/1 -> Math Function1/2
  [D_FS_Local] -> Divide1/1
  Constant4/1 -> Sherwood Number/3
  Constant/1 -> Sherwood Number/1
  Divide1/1 -> Product/2
  Math Function1/1 -> Sherwood Number/4
  Schmidt Number/1(Sc) -> Math Function1/1
  Math Function/1 -> Sherwood Number/2
  Sherwood Number/1 -> Product/1
  Product/1 -> k_m_b/1
  Reynolds Number/1(Re) -> Math Function/1
  Schmidt Number1/1(Sc) -> [Sc_FC_Local]
  Reynolds Number1/1(Re) -> Display/1, [Re_FC_Local]
  U/1 -> Reynolds Number1/1(Flow_Velocity [m/s]), Reynolds Number/1(Flow_Velocity)
  [Rho_FS_Local] -> Reynolds Number1/2(rho [kg/m^3])
  [Mu_FS_Local] -> Reynolds Number1/3(mu [Pa s])
  [Mu_FS_Local] -> Schmidt Number1/1(mu [Pa s])
  [Rho_FS_Local] -> Schmidt Number1/2(rho [kg/m^3])
  [D_FS_Local] -> Schmidt Number1/3(D [m^2/s])
  [Mu_FS_Local] -> Schmidt Number/1(mu)
  [Rho_FS_Local] -> Schmidt Number/2(rho)
  [D_FS_Local] -> Schmidt Number/3(D)
  [Mu_FS_Local] -> Reynolds Number/2(mu)
  [Rho_FS_Local] -> Reynolds Number/3(rho)
  r/1 -> Reynolds Number/4(L)
  T/1 -> Mass Diffusion Coeffecient [m^2 /s]/2(T_Salt [k]), Viscosity W Scaling1/1(T_Salt [k]), Density W Scaling1/1(T_Salt [k])
  Density W Scaling1/1(rho_FS [kg/m^3]) -> [Rho_FS_Local]
  Viscosity W Scaling1/1(mu [Pa-s]) -> Mass Diffusion Coeffecient [m^2 /s]/1(Mu), [Mu_FS_Local]
  Mass Diffusion Coeffecient [m^2 /s]/1(D [m^2/s]) -> [D_FS_Local]

== system Xe_Model_Redo_June_26/Bubbles/Bubble Mass Transfer/Bubble Total KMA/KMA_IC/R2/R2  CV Area ==
  Node Vol. : Inport
  Node T : Inport  Port=2
  CV Vol to Mass Transfer Area1 : Subsystem
  Calc CV Vol W Temp : Subsystem
  A : Outport
  wires:
  CV Vol to Mass Transfer Area1/1(A) -> A/1
  Node T/1 -> Calc CV Vol W Temp/2(T)
  Node Vol./1 -> Calc CV Vol W Temp/1(Vol. Gas)
  Calc CV Vol W Temp/1(V Gas) -> CV Vol to Mass Transfer Area1/1(V)
